simulink model "LKAS_AutoSave_DF_20211126_SW5"  (R2018b)
settings: Solver=FixedStepDiscrete  StartTime=0.0  StopTime=10.0  FixedStep=0.01  RelTol=1e-3
undefined symbols (not defined in the file): LKA_CarWidth, LKA_SampleTime, LKA_StrRatio_C, LKA_Veh2CamL_C, LKA_Veh2CamW_C, LKA_WhlBaseL_C, LL_CompSWA_C, LL_CrvtPrvwT_C, LL_DesDvt_C, LL_DvtComp_C, LL_DvtPrvwT_C, LL_DvtSpdDet_vDvtSpdMin_C, LL_HdAgExT_C, LL_HdAgPrvwT_C, LL_LAccMax_C, LL_LAccRMax_C, LL_LDW_EarliestWarnLine_C, LL_LDW_LatestWarnLine_C, LL_LDWS_SUPPRESS_HEADING, LL_LFClb_TFC_FfCtlRatio_C, LL_LFClb_TFC_KdBalance_C, LL_LFClb_TFC_KdMaxSWA_C, LL_LFClb_TFC_KdV1_C, LL_LFClb_TFC_KdV2_C, LL_LFClb_TFC_KdVehSpdLwr_C, LL_LFClb_TFC_KdVehSpdUpr_C, LL_LFClb_TFC_Ki_C, LL_LFClb_TFC_KiMaxSWA_C, LL_LFClb_TFC_Kp_C, LL_LFClb_TFC_KpKlat_C, LL_LFClb_TFC_KpV1_C, LL_LFClb_TFC_KpV2_C, LL_LFClb_TFC_KpVehSpdLwr_C, LL_LFClb_TFC_KpVehSpdUpr_C, LL_LFClb_TFC_PrvwT_C, LL_LKA_EarliestWarnLine_C, LL_LKA_LatestWarnLine_C, LL_LKAExPrcs_ExitC0Dvt, LL_LKAExPrcs_ExitC0Swt, LL_LKAExPrcs_tiExitTime1, LL_LKAExPrcs_tiExitTime2, LL_LKAExPrcs_tiExitTime3, LL_LKAS_OUT_OF_CONTROL_LAT_VEL, LL_LKAS_OUT_OF_CONTROL_TTLC, LL_LKASWASyn_M0, LL_LKASWASyn_M1, LL_LKASWASyn_M2, LL_LKASWASyn_M3K, LL_LKASWASyn_SWAaddMax, LL_LKASWASyn_T2, LL_LKASWASyn_tiTrqSwaRtTime, LL_LKASWASyn_tiTrqSwaTime, LL_LKASWASyn_TrqMax, LL_LKASWASyn_TrqSwaAddSwt, LL_LKASWASyn_TrqSwaRateDiff, LL_LSpdCompT_C, LL_lStpLngth_C, LL_MAX_DELAY_EPSSTAR_TIME, LL_MAX_DRIVER_TORQUE_DISABLE, LL_MAX_DRIVER_TORQUE_ENABLE ... (+38)
libraries: simulink x137, canmsglib x10, dspstat3 x3, simulink_extras x1
(part 1 of 13)
settings Model: Creator=hejr  LastModifiedBy=hejr
settings OptimizationCC: BlockReduction=off  DefaultParameterBehavior=Inlined  UseDivisionForNetSlopeComputation=on  UseFloatMulNetSlope=on  DefaultUnderspecifiedDataType=single  UseSpecifiedMinMax=on  InlineInvariantSignals=on  PassReuseOutputArgsAs=Individual arguments  ZeroExternalMemoryAtStartup=off  ZeroInternalMemoryAtStartup=off  NoFixptDivByZeroProtection=on  EfficientFloat2IntCast=on  LifeSpan=inf  OptimizeBlockOrder=speed  DifferentSizesBufferReuse=on
settings DebuggingCC: SignalInfNanChecking=error  ReadBeforeWriteMsg=EnableAllAsError  WriteAfterWriteMsg=EnableAllAsError  WriteAfterReadMsg=EnableAllAsError  IntegerOverflowMsg=error  ParameterTunabilityLossMsg=error  UniqueDataStoreMsg=error  AssertControl=DisableAll  NonBusSignalsTreatedAsBus=error  SFInvalidInputDataAccessInChartInitDiag=error  SFTransitionOutsideNaturalParentDiag=error  SFUnreachableExecutionPathDiag=error  SFUndirectedBroadcastEventsDiag=error  IntegerSaturationMsg=error
settings HardwareCC: ProdLongLongMode=on
settings ModelReferenceCC: UpdateModelReferenceTargets=IfOutOfDate
settings SFSimCC: SFSimEcho=off  CompileTimeRecursionLimit=0  EnableRuntimeRecursion=off  MATLABDynamicMemAlloc=off
settings RTWCC: SystemTargetFile=autosar.tlc  GenCodeOnly=on  TemplateMakefile=ert_default_tmf  Description=AUTOSAR  GenerateReport=on  BuildConfiguration=Faster Runs  IncludeHyperlinkInReport=on  LaunchReport=on  GenerateTraceInfo=on  GenerateTraceReport=on  GenerateTraceReportSl=on  GenerateTraceReportSf=on  GenerateTraceReportEml=on  GenerateCodeMetricsReport=on  GenerateCodeReplacementReport=on
settings CodeAppCC: ForceParamTrailComments=on  IgnoreCustomStorageClasses=off  OperatorAnnotations=on  SimulinkDataObjDesc=on  SFDataObjDesc=on  MATLABFcnDesc=on  InsertBlockDesc=on  StateflowObjectComments=on  MATLABSourceComments=on  EnableCustomComments=on  ReqsInCode=on
settings STFCustomTargetCC: TargetLangStandard=C99 (ISO)  MultiwordLength=256  ParMdlRefBuildCompliant=on  CompOptLevelCompliant=on  IncludeMdlTerminateFcn=off  CombineOutputUpdateFcns=on  CombineSignalStateStructs=on  SuppressErrorStatus=on  ERTCustomFileBanners=on  SupportNonFinite=off  SupportComplex=off  SupportContinuousTime=off  SupportNonInlinedSFcns=off  RemoveResetFunc=on  ParenthesesLevel=Maximum  CastingMode=Standards  MATLABClassNameForMDSCustomization=Simulink.SoftwareTarget.ERTCustomization  AutosarCompliant=on  UseToolchainInfoCompliant=on  LookupTableObjectStructAxisOrder=2,1,3,4,...  LUTObjectStructOrderEvenSpacing=Size,Table,Breakpoints  SystemTargetFile=autosar.tlc
settings ERTTargetCC: TargetLangStandard=C99 (ISO)  ConcurrentExecutionCompliant=off  IncludeMdlTerminateFcn=off  CombineSignalStateStructs=on  SuppressErrorStatus=on  SupportNonFinite=off  SupportComplex=off  ParenthesesLevel=Maximum  CastingMode=Standards  ModelStepFunctionPrototypeControlCompliant=off  CPPClassGenCompliant=off  AutosarCompliant=on  LookupTableObjectStructAxisOrder=2,1,3,4,...  LUTObjectStructOrderEvenSpacing=Size,Table,Breakpoints  GenerateASAP2=on  InlinedParameterPlacement=NonHierarchical  ERTCustomFileTemplate=example_file_process.tlc  EnableSignedLeftShifts=off  EnableSignedRightShifts=off

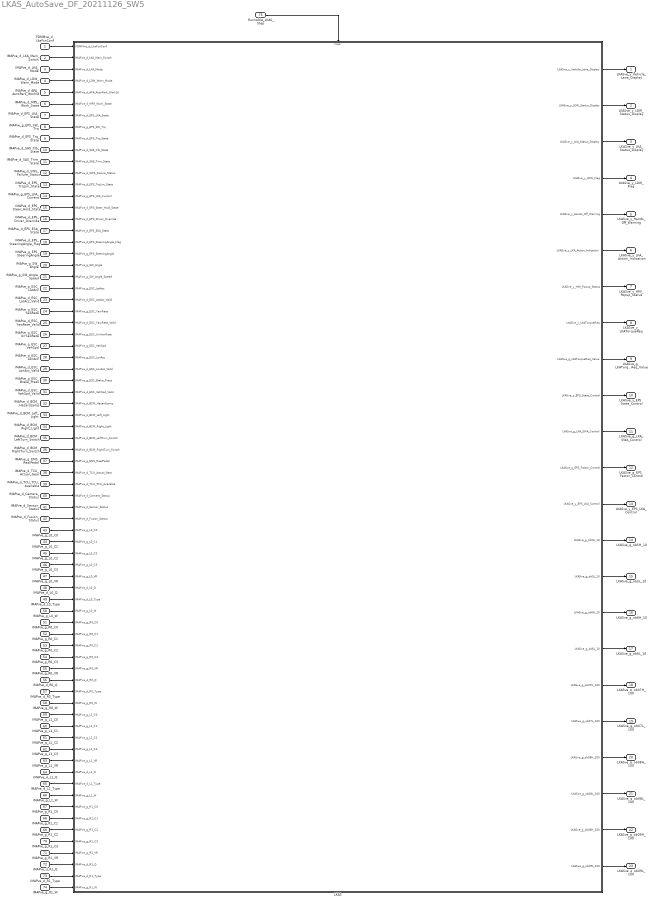
== system LKAS_AutoSave_DF_20211126_SW5 ==
  FDMMve_d_LkaFcnConf : Inport  OutDataTypeStr=UInt16  PortDimensions=1
  IMAPve_d_LKA_Main_Switch : Inport  Port=2  OutDataTypeStr=UInt16  PortDimensions=1
  IMAPve_d_LKA_Mode : Inport  Port=3  OutDataTypeStr=UInt16  PortDimensions=1
  IMAPve_d_LDW_Warn_Mode : Inport  Port=4  OutDataTypeStr=UInt16  PortDimensions=1
  IMAPve_d_APA_AutoPark_WorkSt : Inport  Port=5  OutDataTypeStr=UInt16  PortDimensions=1
  IMAPve_d_MP5_Work_State : Inport  Port=6  OutDataTypeStr=UInt16  PortDimensions=1
  IMAPve_d_EPS_LKA_State : Inport  Port=7  OutDataTypeStr=UInt16  PortDimensions=1
  IMAPve_g_EPS_SW_Trq : Inport  Port=8  OutDataTypeStr=T_M_Nm_Float32  PortDimensions=1
  IMAPve_d_EPS_Trq_State : Inport  Port=9  OutDataTypeStr=UInt16  PortDimensions=1
  IMAPve_d_SAS_Clb_State : Inport  Port=10  OutDataTypeStr=UInt16  PortDimensions=1
  IMAPve_d_SAS_Trim_State : Inport  Port=11  OutDataTypeStr=UInt16  PortDimensions=1
  IMAPve_d_SWS_Failure_Status : Inport  Port=12  OutDataTypeStr=UInt16  PortDimensions=1
  IMAPve_d_EPS_TrqLim_State : Inport  Port=13  OutDataTypeStr=UInt16  PortDimensions=1
  IMAPve_g_EPS_LKA_Current : Inport  Port=14  OutDataTypeStr=T_M_Nm_Float32  PortDimensions=1
  IMAPve_d_EPS_Steer_Hold_State : Inport  Port=15  OutDataTypeStr=UInt16  PortDimensions=1
  IMAPve_d_EPS_Driver_Override : Inport  Port=16  OutDataTypeStr=UInt16  PortDimensions=1
  IMAPve_d_EPS_ESA_State : Inport  Port=17  OutDataTypeStr=UInt16  PortDimensions=1
  IMAPve_d_EPS_SteeringAngle_Flag : Inport  Port=18  OutDataTypeStr=UInt16  PortDimensions=1
  IMAPve_g_EPS_SteeringAngle : Inport  Port=19  OutDataTypeStr=T_M_Nm_Float32  PortDimensions=1
  IMAPve_g_SW_Angle : Inport  Port=20  OutDataTypeStr=T_M_Nm_Float32  PortDimensions=1
  IMAPve_g_SW_Angle_Speed : Inport  Port=21  OutDataTypeStr=T_M_Nm_Float32  PortDimensions=1
  IMAPve_g_ESC_LatAcc : Inport  Port=22  OutDataTypeStr=T_M_Nm_Float32  PortDimensions=1
  IMAPve_d_ESC_LatAcc_Valid : Inport  Port=23  OutDataTypeStr=UInt16  PortDimensions=1
  IMAPve_g_ESC_YawRate : Inport  Port=24  OutDataTypeStr=T_M_Nm_Float32  PortDimensions=1
  IMAPve_d_ESC_YawRate_Valid : Inport  Port=25  OutDataTypeStr=UInt16  PortDimensions=1
  IMAPve_g_ESC_UnYawRate : Inport  Port=26  OutDataTypeStr=T_M_Nm_Float32  PortDimensions=1
  IMAPve_g_ESC_VehSpd : Inport  Port=27  OutDataTypeStr=T_M_Nm_Float32  PortDimensions=1
  IMAPve_g_ESC_LonAcc : Inport  Port=28  OutDataTypeStr=T_M_Nm_Float32  PortDimensions=1
  IMAPve_d_ESC_LonAcc_Valid : Inport  Port=29  OutDataTypeStr=UInt16  PortDimensions=1
  IMAPve_g_ESC_Brake_Press : Inport  Port=30  OutDataTypeStr=T_M_Nm_Float32  PortDimensions=1
  IMAPve_d_ESC_VehSpd_Valid : Inport  Port=31  OutDataTypeStr=UInt16  PortDimensions=1
  IMAPve_d_BCM_HazardLamp : Inport  Port=32  OutDataTypeStr=UInt16  PortDimensions=1
  IMAPve_d_BCM_Left_Light : Inport  Port=33  OutDataTypeStr=UInt16  PortDimensions=1
  IMAPve_d_BCM_Right_Light : Inport  Port=34  OutDataTypeStr=UInt16  PortDimensions=1
  IMAPve_d_BCM_LeftTurn_Switch : Inport  Port=35  OutDataTypeStr=UInt16  PortDimensions=1
  IMAPve_d_BCM_RightTurn_Switch : Inport  Port=36  OutDataTypeStr=UInt16  PortDimensions=1
  IMAPve_g_EMS_RealPedal : Inport  Port=37  OutDataTypeStr=T_M_Nm_Float32  PortDimensions=1
  IMAPve_d_TCU_Actual_Gear : Inport  Port=38  OutDataTypeStr=UInt16  PortDimensions=1
  IMAPve_d_TCU_TCU_Available : Inport  Port=39  OutDataTypeStr=UInt16  PortDimensions=1
  IMAPve_d_Camera_Status : Inport  Port=40  OutDataTypeStr=UInt16  PortDimensions=1
  IMAPve_d_Sensor_Status : Inport  Port=41  OutDataTypeStr=UInt16  PortDimensions=1
  IMAPve_d_Fusion_Status : Inport  Port=42  OutDataTypeStr=UInt16  PortDimensions=1
  IMAPve_g_L0_C0 : Inport  Port=43  OutDataTypeStr=T_M_Nm_Float32  PortDimensions=1
  IMAPve_g_L0_C1 : Inport  Port=44  OutDataTypeStr=T_M_Nm_Float32  PortDimensions=1
  IMAPve_g_L0_C2 : Inport  Port=45  OutDataTypeStr=T_M_Nm_Float32  PortDimensions=1
  IMAPve_g_L0_C3 : Inport  Port=46  OutDataTypeStr=T_M_Nm_Float32  PortDimensions=1
  IMAPve_g_L0_VR : Inport  Port=47  OutDataTypeStr=T_M_Nm_Float32  PortDimensions=1
  IMAPve_d_L0_Q : Inport  Port=48  OutDataTypeStr=UInt16  PortDimensions=1
  IMAPve_d_L0_Type : Inport  Port=49  OutDataTypeStr=UInt16  PortDimensions=1
  IMAPve_g_L0_W : Inport  Port=50  OutDataTypeStr=T_M_Nm_Float32  PortDimensions=1
  IMAPve_g_R0_C0 : Inport  Port=51  OutDataTypeStr=T_M_Nm_Float32  PortDimensions=1
  IMAPve_g_R0_C1 : Inport  Port=52  OutDataTypeStr=T_M_Nm_Float32  PortDimensions=1
  IMAPve_g_R0_C2 : Inport  Port=53  OutDataTypeStr=T_M_Nm_Float32  PortDimensions=1
  IMAPve_g_R0_C3 : Inport  Port=54  OutDataTypeStr=T_M_Nm_Float32  PortDimensions=1
  IMAPve_g_R0_VR : Inport  Port=55  OutDataTypeStr=T_M_Nm_Float32  PortDimensions=1
  IMAPve_d_R0_Q : Inport  Port=56  OutDataTypeStr=UInt16  PortDimensions=1
  IMAPve_d_R0_Type : Inport  Port=57  OutDataTypeStr=UInt16  PortDimensions=1
  IMAPve_g_R0_W : Inport  Port=58  OutDataTypeStr=T_M_Nm_Float32  PortDimensions=1
  IMAPve_g_L1_C0 : Inport  Port=59  OutDataTypeStr=T_M_Nm_Float32  PortDimensions=1
  IMAPve_g_L1_C1 : Inport  Port=60  OutDataTypeStr=T_M_Nm_Float32  PortDimensions=1
  IMAPve_g_L1_C2 : Inport  Port=61  OutDataTypeStr=T_M_Nm_Float32  PortDimensions=1
  IMAPve_g_L1_C3 : Inport  Port=62  OutDataTypeStr=T_M_Nm_Float32  PortDimensions=1
  IMAPve_g_L1_VR : Inport  Port=63  OutDataTypeStr=T_M_Nm_Float32  PortDimensions=1
  IMAPve_d_L1_Q : Inport  Port=64  OutDataTypeStr=UInt16  PortDimensions=1
  IMAPve_d_L1_Type : Inport  Port=65  OutDataTypeStr=UInt16  PortDimensions=1
  IMAPve_g_L1_W : Inport  Port=66  OutDataTypeStr=T_M_Nm_Float32  PortDimensions=1
  IMAPve_g_R1_C0 : Inport  Port=67  OutDataTypeStr=T_M_Nm_Float32  PortDimensions=1
  IMAPve_g_R1_C1 : Inport  Port=68  OutDataTypeStr=T_M_Nm_Float32  PortDimensions=1
  IMAPve_g_R1_C2 : Inport  Port=69  OutDataTypeStr=T_M_Nm_Float32  PortDimensions=1
  IMAPve_g_R1_C3 : Inport  Port=70  OutDataTypeStr=T_M_Nm_Float32  PortDimensions=1
  IMAPve_g_R1_VR : Inport  Port=71  OutDataTypeStr=T_M_Nm_Float32  PortDimensions=1
  IMAPve_d_R1_Q : Inport  Port=72  OutDataTypeStr=UInt16  PortDimensions=1
  IMAPve_d_R1_Type : Inport  Port=73  OutDataTypeStr=UInt16  PortDimensions=1
  IMAPve_g_R1_W : Inport  Port=74  OutDataTypeStr=T_M_Nm_Float32  PortDimensions=1
  Runnable_LKAS_Step : Inport  Port=75  SampleTime=0.01  OutputFunctionCall=on
  LKAS : Subsystem  TreatAsAtomicUnit=on
  LKASve_y_Vehicle_Lane_Display : Outport  OutDataTypeStr=UInt8  PortDimensions=1
  LKASve_y_LDW_Status_Display : Outport  Port=2  OutDataTypeStr=UInt8  PortDimensions=1
  LKASve_y_LKA_Status_Display : Outport  Port=3  OutDataTypeStr=UInt8  PortDimensions=1
  LKASve_y_LDW_Flag : Outport  Port=4  OutDataTypeStr=UInt8  PortDimensions=1
  LKASve_y_Hands_Off_Warning : Outport  Port=5  OutDataTypeStr=UInt8  PortDimensions=1
  LKASve_y_LKA_Action_Indication : Outport  Port=6  OutDataTypeStr=UInt8  PortDimensions=1
  LKASve_y_HMI_Popup_Status : Outport  Port=7  OutDataTypeStr=UInt8  PortDimensions=1
  LKASve_y_LKATorqueReq : Outport  Port=8  OutDataTypeStr=UInt8  PortDimensions=1
  LKASve_g_LKATorqueReq_Value : Outport  Port=9  OutDataTypeStr=T_M_Nm_Float32  PortDimensions=1
  LKASve_y_EPS_State_Control : Outport  Port=10  OutDataTypeStr=UInt8  PortDimensions=1
  LKASve_g_LKA_SWA_Control : Outport  Port=11  OutDataTypeStr=T_M_Nm_Float32  PortDimensions=1
  LKASve_g_EPS_Factor_Control : Outport  Port=12  OutDataTypeStr=T_M_Nm_Float32  PortDimensions=1
  LKASve_y_EPS_LKA_Control : Outport  Port=13  OutDataTypeStr=UInt8  PortDimensions=1
  LKASve_g_ob5H_10 : Outport  Port=14  OutDataTypeStr=UInt32  PortDimensions=1
  LKASve_g_ob5L_10 : Outport  Port=15  OutDataTypeStr=UInt32  PortDimensions=1
  LKASve_g_ob6H_10 : Outport  Port=16  OutDataTypeStr=UInt32  PortDimensions=1
  LKASve_g_ob6L_10 : Outport  Port=17  OutDataTypeStr=UInt32  PortDimensions=1
  LKASve_g_ob07H_100 : Outport  Port=18  OutDataTypeStr=UInt32  PortDimensions=1
  LKASve_g_ob07L_100 : Outport  Port=19  OutDataTypeStr=UInt32  PortDimensions=1
  LKASve_g_ob08H_100 : Outport  Port=20  OutDataTypeStr=UInt32  PortDimensions=1
  LKASve_g_ob08L_100 : Outport  Port=21  OutDataTypeStr=UInt32  PortDimensions=1
  LKASve_g_ob09H_100 : Outport  Port=22  OutDataTypeStr=UInt32  PortDimensions=1
  LKASve_g_ob09L_100 : Outport  Port=23  OutDataTypeStr=UInt32  PortDimensions=1
  wires:
  FDMMve_d_LkaFcnConf/1 -> LKAS/1(FDMMve_d_LkaFcnConf)
  IMAPve_d_LKA_Main_Switch/1 -> LKAS/2(IMAPve_d_LKA_Main_Switch)
  IMAPve_d_LKA_Mode/1 -> LKAS/3(IMAPve_d_LKA_Mode)
  IMAPve_d_LDW_Warn_Mode/1 -> LKAS/4(IMAPve_d_LDW_Warn_Mode)
  IMAPve_d_APA_AutoPark_WorkSt/1 -> LKAS/5(IMAPve_d_APA_AutoPark_WorkSt)
  IMAPve_d_MP5_Work_State/1 -> LKAS/6(IMAPve_d_MP5_Work_State)
  IMAPve_d_EPS_LKA_State/1 -> LKAS/7(IMAPve_d_EPS_LKA_State)
  IMAPve_g_EPS_SW_Trq/1 -> LKAS/8(IMAPve_g_EPS_SW_Trq)
  IMAPve_d_EPS_Trq_State/1 -> LKAS/9(IMAPve_d_EPS_Trq_State)
  IMAPve_d_SAS_Clb_State/1 -> LKAS/10(IMAPve_d_SAS_Clb_State)
  IMAPve_d_SAS_Trim_State/1 -> LKAS/11(IMAPve_d_SAS_Trim_State)
  IMAPve_d_SWS_Failure_Status/1 -> LKAS/12(IMAPve_d_SWS_Failure_Status)
  IMAPve_d_EPS_TrqLim_State/1 -> LKAS/13(IMAPve_d_EPS_TrqLim_State)
  IMAPve_g_EPS_LKA_Current/1 -> LKAS/14(IMAPve_g_EPS_LKA_Current)
  IMAPve_d_EPS_Steer_Hold_State/1 -> LKAS/15(IMAPve_d_EPS_Steer_Hold_State)
  IMAPve_d_EPS_Driver_Override/1 -> LKAS/16(IMAPve_d_EPS_Driver_Override)
  IMAPve_d_EPS_ESA_State/1 -> LKAS/17(IMAPve_d_EPS_ESA_State)
  IMAPve_d_EPS_SteeringAngle_Flag/1 -> LKAS/18(IMAPve_d_EPS_SteeringAngle_Flag)
  IMAPve_g_EPS_SteeringAngle/1 -> LKAS/19(IMAPve_g_EPS_SteeringAngle)
  IMAPve_g_SW_Angle/1 -> LKAS/20(IMAPve_g_SW_Angle)
  IMAPve_g_SW_Angle_Speed/1 -> LKAS/21(IMAPve_g_SW_Angle_Speed)
  IMAPve_g_ESC_LatAcc/1 -> LKAS/22(IMAPve_g_ESC_LatAcc)
  IMAPve_d_ESC_LatAcc_Valid/1 -> LKAS/23(IMAPve_d_ESC_LatAcc_Valid)
  IMAPve_g_ESC_YawRate/1 -> LKAS/24(IMAPve_g_ESC_YawRate)
  IMAPve_d_ESC_YawRate_Valid/1 -> LKAS/25(IMAPve_d_ESC_YawRate_Valid)
  IMAPve_g_ESC_UnYawRate/1 -> LKAS/26(IMAPve_g_ESC_UnYawRate)
  IMAPve_g_ESC_VehSpd/1 -> LKAS/27(IMAPve_g_ESC_VehSpd)
  IMAPve_g_ESC_LonAcc/1 -> LKAS/28(IMAPve_g_ESC_LonAcc)
  IMAPve_d_ESC_LonAcc_Valid/1 -> LKAS/29(IMAPve_d_ESC_LonAcc_Valid)
  IMAPve_g_ESC_Brake_Press/1 -> LKAS/30(IMAPve_g_ESC_Brake_Press)
  IMAPve_d_ESC_VehSpd_Valid/1 -> LKAS/31(IMAPve_d_ESC_VehSpd_Valid)
  IMAPve_d_BCM_HazardLamp/1 -> LKAS/32(IMAPve_d_BCM_HazardLamp)
  IMAPve_d_BCM_Left_Light/1 -> LKAS/33(IMAPve_d_BCM_Left_Light)
  IMAPve_d_BCM_Right_Light/1 -> LKAS/34(IMAPve_d_BCM_Right_Light)
  IMAPve_d_BCM_LeftTurn_Switch/1 -> LKAS/35(IMAPve_d_BCM_LeftTurn_Switch)
  IMAPve_d_BCM_RightTurn_Switch/1 -> LKAS/36(IMAPve_d_BCM_RightTurn_Switch)
  IMAPve_g_EMS_RealPedal/1 -> LKAS/37(IMAPve_g_EMS_RealPedal)
  IMAPve_d_TCU_Actual_Gear/1 -> LKAS/38(IMAPve_d_TCU_Actual_Gear)
  IMAPve_d_TCU_TCU_Available/1 -> LKAS/39(IMAPve_d_TCU_TCU_Available)
  IMAPve_d_Camera_Status/1 -> LKAS/40(IMAPve_d_Camera_Status)
  IMAPve_d_Sensor_Status/1 -> LKAS/41(IMAPve_d_Sensor_Status)
  IMAPve_d_Fusion_Status/1 -> LKAS/42(IMAPve_d_Fusion_Status)
  IMAPve_g_L0_C0/1 -> LKAS/43(IMAPve_g_L0_C0)
  IMAPve_g_L0_C1/1 -> LKAS/44(IMAPve_g_L0_C1)
  IMAPve_g_L0_C2/1 -> LKAS/45(IMAPve_g_L0_C2)
  IMAPve_g_L0_C3/1 -> LKAS/46(IMAPve_g_L0_C3)
  IMAPve_g_L0_VR/1 -> LKAS/47(IMAPve_g_L0_VR)
  IMAPve_d_L0_Q/1 -> LKAS/48(IMAPve_d_L0_Q)
  IMAPve_d_L0_Type/1 -> LKAS/49(IMAPve_d_L0_Type)
  IMAPve_g_L0_W/1 -> LKAS/50(IMAPve_g_L0_W)
  IMAPve_g_R0_C0/1 -> LKAS/51(IMAPve_g_R0_C0)
  IMAPve_g_R0_C1/1 -> LKAS/52(IMAPve_g_R0_C1)
  IMAPve_g_R0_C2/1 -> LKAS/53(IMAPve_g_R0_C2)
  IMAPve_g_R0_C3/1 -> LKAS/54(IMAPve_g_R0_C3)
  IMAPve_g_R0_VR/1 -> LKAS/55(IMAPve_g_R0_VR)
  IMAPve_d_R0_Q/1 -> LKAS/56(IMAPve_d_R0_Q)
  IMAPve_d_R0_Type/1 -> LKAS/57(IMAPve_d_R0_Type)
  IMAPve_g_R0_W/1 -> LKAS/58(IMAPve_g_R0_W)
  IMAPve_g_L1_C0/1 -> LKAS/59(IMAPve_g_L1_C0)
  IMAPve_g_L1_C1/1 -> LKAS/60(IMAPve_g_L1_C1)
  IMAPve_g_L1_C2/1 -> LKAS/61(IMAPve_g_L1_C2)
  IMAPve_g_L1_C3/1 -> LKAS/62(IMAPve_g_L1_C3)
  IMAPve_g_L1_VR/1 -> LKAS/63(IMAPve_g_L1_VR)
  IMAPve_d_L1_Q/1 -> LKAS/64(IMAPve_d_L1_Q)
  IMAPve_d_L1_Type/1 -> LKAS/65(IMAPve_d_L1_Type)
  IMAPve_g_L1_W/1 -> LKAS/66(IMAPve_g_L1_W)
  IMAPve_g_R1_C0/1 -> LKAS/67(IMAPve_g_R1_C0)
  IMAPve_g_R1_C1/1 -> LKAS/68(IMAPve_g_R1_C1)
  IMAPve_g_R1_C2/1 -> LKAS/69(IMAPve_g_R1_C2)
  IMAPve_g_R1_C3/1 -> LKAS/70(IMAPve_g_R1_C3)
  IMAPve_g_R1_VR/1 -> LKAS/71(IMAPve_g_R1_VR)
  IMAPve_d_R1_Q/1 -> LKAS/72(IMAPve_d_R1_Q)
  IMAPve_d_R1_Type/1 -> LKAS/73(IMAPve_d_R1_Type)
  IMAPve_g_R1_W/1 -> LKAS/74(IMAPve_g_R1_W)
  Runnable_LKAS_Step/1 -> LKAS/Trigger
  LKAS/1(LKASve_y_Vehicle_Lane_Display) -> LKASve_y_Vehicle_Lane_Display/1
  LKAS/2(LKASve_y_LDW_Status_Display) -> LKASve_y_LDW_Status_Display/1
  LKAS/3(LKASve_y_LKA_Status_Display) -> LKASve_y_LKA_Status_Display/1
  LKAS/4(LKASve_y_LDW_Flag) -> LKASve_y_LDW_Flag/1
  LKAS/5(LKASve_y_Hands_Off_Warning) -> LKASve_y_Hands_Off_Warning/1
  LKAS/6(LKASve_y_LKA_Action_Indication) -> LKASve_y_LKA_Action_Indication/1
  LKAS/7(LKASve_y_HMI_Popup_Status) -> LKASve_y_HMI_Popup_Status/1
  LKAS/8(LKASve_y_LKATorqueReq) -> LKASve_y_LKATorqueReq/1
  LKAS/9(LKASve_g_LKATorqueReq_Value) -> LKASve_g_LKATorqueReq_Value/1
  LKAS/10(LKASve_y_EPS_State_Control) -> LKASve_y_EPS_State_Control/1
  LKAS/11(LKASve_g_LKA_SWA_Control) -> LKASve_g_LKA_SWA_Control/1
  LKAS/12(LKASve_g_EPS_Factor_Control) -> LKASve_g_EPS_Factor_Control/1
  LKAS/13(LKASve_y_EPS_LKA_Control) -> LKASve_y_EPS_LKA_Control/1
  LKAS/14(LKASve_g_ob5H_10) -> LKASve_g_ob5H_10/1
  LKAS/15(LKASve_g_ob5L_10) -> LKASve_g_ob5L_10/1
  LKAS/16(LKASve_g_ob6H_10) -> LKASve_g_ob6H_10/1
  LKAS/17(LKASve_g_ob6L_10) -> LKASve_g_ob6L_10/1
  LKAS/18(LKASve_g_ob07H_100) -> LKASve_g_ob07H_100/1
  LKAS/19(LKASve_g_ob07L_100) -> LKASve_g_ob07L_100/1
  LKAS/20(LKASve_g_ob08H_100) -> LKASve_g_ob08H_100/1
  LKAS/21(LKASve_g_ob08L_100) -> LKASve_g_ob08L_100/1
  LKAS/22(LKASve_g_ob09H_100) -> LKASve_g_ob09H_100/1
  LKAS/23(LKASve_g_ob09L_100) -> LKASve_g_ob09L_100/1

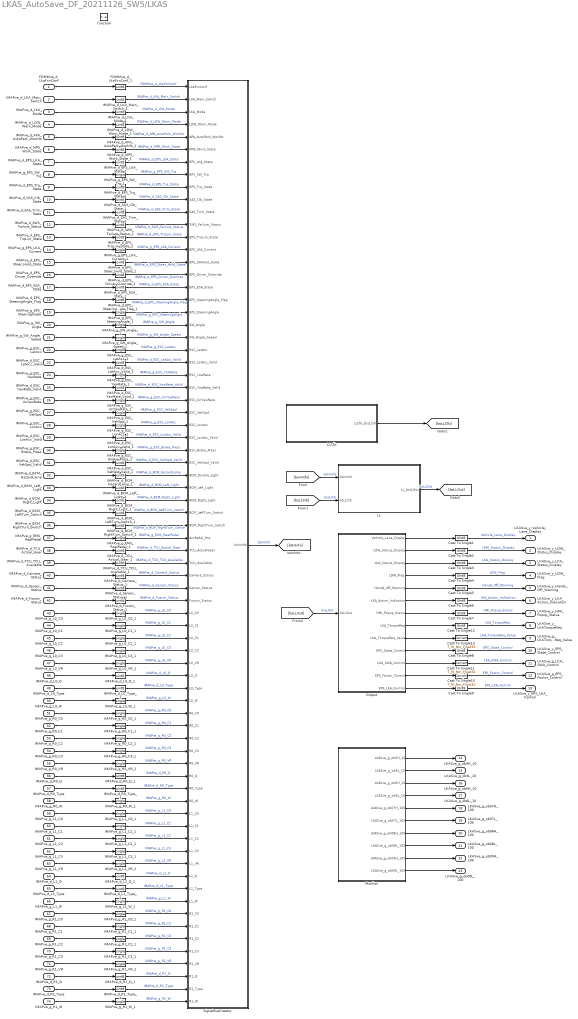
== system LKAS_AutoSave_DF_20211126_SW5/LKAS ==
  FDMMve_d_LkaFcnConf : Inport
  IMAPve_d_LKA_Main_Switch : Inport  Port=2
  IMAPve_d_LKA_Mode : Inport  Port=3
  IMAPve_d_LDW_Warn_Mode : Inport  Port=4
  IMAPve_d_APA_AutoPark_WorkSt : Inport  Port=5
  IMAPve_d_MP5_Work_State : Inport  Port=6
  IMAPve_d_EPS_LKA_State : Inport  Port=7
  IMAPve_g_EPS_SW_Trq : Inport  Port=8
  IMAPve_d_EPS_Trq_State : Inport  Port=9
  IMAPve_d_SAS_Clb_State : Inport  Port=10
  IMAPve_d_SAS_Trim_State : Inport  Port=11
  IMAPve_d_SWS_Failure_Status : Inport  Port=12
  IMAPve_d_EPS_TrqLim_State : Inport  Port=13
  IMAPve_g_EPS_LKA_Current : Inport  Port=14
  IMAPve_d_EPS_Steer_Hold_State : Inport  Port=15
  IMAPve_d_EPS_Driver_Override : Inport  Port=16
  IMAPve_d_EPS_ESA_State : Inport  Port=17
  IMAPve_d_EPS_SteeringAngle_Flag : Inport  Port=18
  IMAPve_g_EPS_SteeringAngle : Inport  Port=19
  IMAPve_g_SW_Angle : Inport  Port=20
  IMAPve_g_SW_Angle_Speed : Inport  Port=21
  IMAPve_g_ESC_LatAcc : Inport  Port=22
  IMAPve_d_ESC_LatAcc_Valid : Inport  Port=23
  IMAPve_g_ESC_YawRate : Inport  Port=24
  IMAPve_d_ESC_YawRate_Valid : Inport  Port=25
  IMAPve_g_ESC_UnYawRate : Inport  Port=26
  IMAPve_g_ESC_VehSpd : Inport  Port=27
  IMAPve_g_ESC_LonAcc : Inport  Port=28
  IMAPve_d_ESC_LonAcc_Valid : Inport  Port=29
  IMAPve_g_ESC_Brake_Press : Inport  Port=30
  IMAPve_d_ESC_VehSpd_Valid : Inport  Port=31
  IMAPve_d_BCM_HazardLamp : Inport  Port=32
  IMAPve_d_BCM_Left_Light : Inport  Port=33
  IMAPve_d_BCM_Right_Light : Inport  Port=34
  IMAPve_d_BCM_LeftTurn_Switch : Inport  Port=35
  IMAPve_d_BCM_RightTurn_Switch : Inport  Port=36
  IMAPve_g_EMS_RealPedal : Inport  Port=37
  IMAPve_d_TCU_Actual_Gear : Inport  Port=38
  IMAPve_d_TCU_TCU_Available : Inport  Port=39
  IMAPve_d_Camera_Status : Inport  Port=40
  IMAPve_d_Sensor_Status : Inport  Port=41
  IMAPve_d_Fusion_Status : Inport  Port=42
  IMAPve_g_L0_C0 : Inport  Port=43
  IMAPve_g_L0_C1 : Inport  Port=44
  IMAPve_g_L0_C2 : Inport  Port=45
  IMAPve_g_L0_C3 : Inport  Port=46
  IMAPve_g_L0_VR : Inport  Port=47
  IMAPve_d_L0_Q : Inport  Port=48
  IMAPve_d_L0_Type : Inport  Port=49
  IMAPve_g_L0_W : Inport  Port=50
  IMAPve_g_R0_C0 : Inport  Port=51
  IMAPve_g_R0_C1 : Inport  Port=52
  IMAPve_g_R0_C2 : Inport  Port=53
  IMAPve_g_R0_C3 : Inport  Port=54
  IMAPve_g_R0_VR : Inport  Port=55
  IMAPve_d_R0_Q : Inport  Port=56
  IMAPve_d_R0_Type : Inport  Port=57
  IMAPve_g_R0_W : Inport  Port=58
  IMAPve_g_L1_C0 : Inport  Port=59
  IMAPve_g_L1_C1 : Inport  Port=60
  IMAPve_g_L1_C2 : Inport  Port=61
  IMAPve_g_L1_C3 : Inport  Port=62
  IMAPve_g_L1_VR : Inport  Port=63
  IMAPve_d_L1_Q : Inport  Port=64
  IMAPve_d_L1_Type : Inport  Port=65
  IMAPve_g_L1_W : Inport  Port=66
  IMAPve_g_R1_C0 : Inport  Port=67
  IMAPve_g_R1_C1 : Inport  Port=68
  IMAPve_g_R1_C2 : Inport  Port=69
  IMAPve_g_R1_C3 : Inport  Port=70
  IMAPve_g_R1_VR : Inport  Port=71
  IMAPve_d_R1_Q : Inport  Port=72
  IMAPve_d_R1_Type : Inport  Port=73
  IMAPve_g_R1_W : Inport  Port=74
  function : TriggerPort  TriggerType=function-call  VariantControl=Variant  SampleTimeType=periodic  SampleTime=-1
  Cast To Single{1..9,12} (10 alike) : DataTypeConversion  OutDataTypeStr=UInt8
  Cast To Single10 : DataTypeConversion  OutDataTypeStr=T_M_Nm_Float32
  Cast To Single11 : DataTypeConversion  OutDataTypeStr=T_M_Nm_Float32
  Cast To Single13 : DataTypeConversion  OutDataTypeStr=T_M_Nm_Float32
  FDMMve_d_LkaFcnConf_1 : DataTypeConversion  OutDataTypeStr=uint8
  IMAPve_d_APA_AutoPark_WorkSt_1 : DataTypeConversion  OutDataTypeStr=uint8
  IMAPve_d_BCM_HazardLamp_1 : DataTypeConversion  OutDataTypeStr=uint8
  IMAPve_d_BCM_LeftTurn_Switch_1 : DataTypeConversion  OutDataTypeStr=uint8
  IMAPve_d_BCM_Left_Light_1 : DataTypeConversion  OutDataTypeStr=uint8
  IMAPve_d_BCM_RightTurn_Switch_1 : DataTypeConversion  OutDataTypeStr=uint8
  IMAPve_d_BCM_Right_Light_1 : DataTypeConversion  OutDataTypeStr=uint8
  IMAPve_d_Camera_Status_1 : DataTypeConversion  OutDataTypeStr=uint8
  IMAPve_d_EPS_Driver_Override_1 : DataTypeConversion  OutDataTypeStr=uint8
  IMAPve_d_EPS_ESA_State_1 : DataTypeConversion  OutDataTypeStr=uint8
  IMAPve_d_EPS_LKA_State_1 : DataTypeConversion  OutDataTypeStr=uint8
  IMAPve_d_EPS_Steer_Hold_State_1 : DataTypeConversion  OutDataTypeStr=uint8
  IMAPve_d_EPS_SteeringAngle_Flag_1 : DataTypeConversion  OutDataTypeStr=uint8
  IMAPve_d_EPS_TrqLim_State_1 : DataTypeConversion  OutDataTypeStr=uint8
  IMAPve_d_EPS_Trq_State_1 : DataTypeConversion  OutDataTypeStr=uint8
  IMAPve_d_ESC_LatAcc_Valid_1 : DataTypeConversion  OutDataTypeStr=uint8
  IMAPve_d_ESC_LonAcc_Valid_1 : DataTypeConversion  OutDataTypeStr=uint8
  IMAPve_d_ESC_VehSpd_Valid_1 : DataTypeConversion  OutDataTypeStr=uint8
  IMAPve_d_ESC_YawRate_Valid_1 : DataTypeConversion  OutDataTypeStr=uint8
  IMAPve_d_Fusion_Status_1 : DataTypeConversion  OutDataTypeStr=uint8
  IMAPve_d_L0_Q_1 : DataTypeConversion  OutDataTypeStr=uint8
  IMAPve_d_L0_Type_1 : DataTypeConversion  OutDataTypeStr=uint8
  IMAPve_d_L1_Q_1 : DataTypeConversion  OutDataTypeStr=uint8
  IMAPve_d_L1_Type_1 : DataTypeConversion  OutDataTypeStr=uint8
  IMAPve_d_LDW_Warn_Mode_1 : DataTypeConversion  OutDataTypeStr=uint8
  IMAPve_d_LKA_Main_Switch_1 : DataTypeConversion  OutDataTypeStr=uint8
  IMAPve_d_LKA_Mode_1 : DataTypeConversion  OutDataTypeStr=uint8
  IMAPve_d_MP5_Work_State_1 : DataTypeConversion  OutDataTypeStr=uint8
  IMAPve_d_R0_Q_1 : DataTypeConversion  OutDataTypeStr=uint8
  IMAPve_d_R0_Type_1 : DataTypeConversion  OutDataTypeStr=uint8
  IMAPve_d_R1_Q_1 : DataTypeConversion  OutDataTypeStr=uint8
  IMAPve_d_R1_Type_1 : DataTypeConversion  OutDataTypeStr=uint8
  IMAPve_d_SAS_Clb_State_1 : DataTypeConversion  OutDataTypeStr=uint8
  IMAPve_d_SAS_Trim_State_1 : DataTypeConversion  OutDataTypeStr=uint8
  IMAPve_d_SWS_Failure_Status_1 : DataTypeConversion  OutDataTypeStr=uint8
  IMAPve_d_Sensor_Status_1 : DataTypeConversion  OutDataTypeStr=uint8
  IMAPve_d_TCU_Actual_Gear_1 : DataTypeConversion  OutDataTypeStr=uint8
  IMAPve_d_TCU_TCU_Available_1 : DataTypeConversion  OutDataTypeStr=uint8
  IMAPve_g_EMS_RealPedal_1 : DataTypeConversion  OutDataTypeStr=single
  IMAPve_g_EPS_LKA_Current_1 : DataTypeConversion  OutDataTypeStr=single
  IMAPve_g_EPS_SW_Trq_1 : DataTypeConversion  OutDataTypeStr=single
  IMAPve_g_EPS_SteeringAngle_1 : DataTypeConversion  OutDataTypeStr=single
  IMAPve_g_ESC_Brake_Press_1 : DataTypeConversion  OutDataTypeStr=single
  IMAPve_g_ESC_LatAcc_1 : DataTypeConversion  OutDataTypeStr=single
  IMAPve_g_ESC_LonAcc_1 : DataTypeConversion  OutDataTypeStr=single
  IMAPve_g_ESC_UnYawRate_1 : DataTypeConversion  OutDataTypeStr=single
  IMAPve_g_ESC_VehSpd_1 : DataTypeConversion  OutDataTypeStr=single
  IMAPve_g_ESC_YawRate_1 : DataTypeConversion  OutDataTypeStr=single
  IMAPve_g_L0_C0_1 : DataTypeConversion  OutDataTypeStr=single
  IMAPve_g_L0_C1_1 : DataTypeConversion  OutDataTypeStr=single
  IMAPve_g_L0_C2_1 : DataTypeConversion  OutDataTypeStr=single
  IMAPve_g_L0_C3_1 : DataTypeConversion  OutDataTypeStr=single
  IMAPve_g_L0_VR_1 : DataTypeConversion  OutDataTypeStr=single
  IMAPve_g_L0_W_1 : DataTypeConversion  OutDataTypeStr=single
  IMAPve_g_L1_C0_1 : DataTypeConversion  OutDataTypeStr=single
  IMAPve_g_L1_C1_1 : DataTypeConversion  OutDataTypeStr=single
  IMAPve_g_L1_C2_1 : DataTypeConversion  OutDataTypeStr=single
  IMAPve_g_L1_C3_1 : DataTypeConversion  OutDataTypeStr=single
  IMAPve_g_L1_VR_1 : DataTypeConversion  OutDataTypeStr=single
  IMAPve_g_L1_W_1 : DataTypeConversion  OutDataTypeStr=single
  IMAPve_g_R0_C0_1 : DataTypeConversion  OutDataTypeStr=single
  IMAPve_g_R0_C1_1 : DataTypeConversion  OutDataTypeStr=single
  IMAPve_g_R0_C2_1 : DataTypeConversion  OutDataTypeStr=single
  IMAPve_g_R0_C3_1 : DataTypeConversion  OutDataTypeStr=single
  IMAPve_g_R0_VR_1 : DataTypeConversion  OutDataTypeStr=single
  IMAPve_g_R0_W_1 : DataTypeConversion  OutDataTypeStr=single
  IMAPve_g_R1_C0_1 : DataTypeConversion  OutDataTypeStr=single
  IMAPve_g_R1_C1_1 : DataTypeConversion  OutDataTypeStr=single
  IMAPve_g_R1_C2_1 : DataTypeConversion  OutDataTypeStr=single
  IMAPve_g_R1_C3_1 : DataTypeConversion  OutDataTypeStr=single
  IMAPve_g_R1_VR_1 : DataTypeConversion  OutDataTypeStr=single
  IMAPve_g_R1_W_1 : DataTypeConversion  OutDataTypeStr=single
  IMAPve_g_SW_Angle_1 : DataTypeConversion  OutDataTypeStr=single
  IMAPve_g_SW_Angle_Speed_1 : DataTypeConversion  OutDataTypeStr=single
  LL : Subsystem
  LLClb : Subsystem
  Monitor : Subsystem  SystemSampleTime=0.01
  Output : Subsystem
  SignalBusCreator : Subsystem
  LKASve_y_Vehicle_Lane_Display : Outport
  LKASve_y_LDW_Status_Display : Outport  Port=2
  LKASve_y_LKA_Status_Display : Outport  Port=3
  LKASve_y_LDW_Flag : Outport  Port=4
  LKASve_y_Hands_Off_Warning : Outport  Port=5
  LKASve_y_LKA_Action_Indication : Outport  Port=6
  LKASve_y_HMI_Popup_Status : Outport  Port=7
  LKASve_y_LKATorqueReq : Outport  Port=8
  LKASve_g_LKATorqueReq_Value : Outport  Port=9
  LKASve_y_EPS_State_Control : Outport  Port=10
  LKASve_g_LKA_SWA_Control : Outport  Port=11
  LKASve_g_EPS_Factor_Control : Outport  Port=12
  LKASve_y_EPS_LKA_Control : Outport  Port=13
  LKASve_g_ob5H_10 : Outport  Port=14
  LKASve_g_ob5L_10 : Outport  Port=15
  LKASve_g_ob6H_10 : Outport  Port=16
  LKASve_g_ob6L_10 : Outport  Port=17
  LKASve_g_ob07H_100 : Outport  Port=18
  LKASve_g_ob07L_100 : Outport  Port=19
  LKASve_g_ob08H_100 : Outport  Port=20
  LKASve_g_ob08L_100 : Outport  Port=21
  LKASve_g_ob09H_100 : Outport  Port=22
  LKASve_g_ob09L_100 : Outport  Port=23
  wires:
  Cast To Single9/1 -> LKASve_y_EPS_LKA_Control/1  "EPS_LKA_Control"
  Cast To Single10/1 -> LKASve_g_EPS_Factor_Control/1  "EPS_Factor_Control"
  Cast To Single11/1 -> LKASve_g_LKA_SWA_Control/1  "LKA_SWA_Control"
  Cast To Single8/1 -> LKASve_y_EPS_State_Control/1  "EPS_State_Control"
  Cast To Single13/1 -> LKASve_g_LKATorqueReq_Value/1  "LKA_TorqueReq_Value"
  Cast To Single12/1 -> LKASve_y_LKATorqueReq/1  "LKA_TorqueReq"
  Cast To Single7/1 -> LKASve_y_HMI_Popup_Status/1  "HMI_Popup_Status"
  Cast To Single6/1 -> LKASve_y_LKA_Action_Indication/1  "LKA_Action_Indication"
  Cast To Single5/1 -> LKASve_y_Hands_Off_Warning/1  "Hands_Off_Warning"
  Cast To Single4/1 -> LKASve_y_LDW_Flag/1  "LDW_Flag"
  Cast To Single3/1 -> LKASve_y_LKA_Status_Display/1  "LKA_Status_Display"
  Cast To Single2/1 -> LKASve_y_LDW_Status_Display/1  "LDW_Status_Display"
  Cast To Single1/1 -> LKASve_y_Vehicle_Lane_Display/1  "Vehicle_Lane_Display"
  Output/13(EPS_LKA_Control) -> Cast To Single9/1
  Output/12(EPS_Factor_Control) -> Cast To Single10/1
  Output/11(LKA_SWA_Control) -> Cast To Single11/1
  Output/10(EPS_State_Control) -> Cast To Single8/1
  Output/9(LKA_TorqueReq_Value) -> Cast To Single13/1
  Output/8(LKA_TorqueReq) -> Cast To Single12/1
  Output/7(HMI_Popup_Status) -> Cast To Single7/1
  Output/6(LKA_Action_Indication) -> Cast To Single6/1
  Output/5(Hands_Off_Warning) -> Cast To Single5/1
  Output/4(LDW_Flag) -> Cast To Single4/1
  Output/3(LKA_Status_Display) -> Cast To Single3/1
  Output/2(LDW_Status_Display) -> Cast To Single2/1
  Output/1(Vehicle_Lane_Display) -> Cast To Single1/1
  Monitor/2(LKASve_g_ob5L_10) -> LKASve_g_ob5L_10/1
  [bsInInfo] -> LL/1(bsInInfo)  "bsInInfo"
  Monitor/5(LKASve_g_ob07H_100) -> LKASve_g_ob07H_100/1
  Monitor/10(LKASve_g_ob09L_100) -> LKASve_g_ob09L_100/1
  Monitor/4(LKASve_g_ob6L_10) -> LKASve_g_ob6L_10/1
  SignalBusCreator/1(bsInInfo) -> [bsInInfo]  "bsInInfo"
  LLClb/1(LLClb_bsLLClb) -> [bsLLClb]
  LL/1(LL_bsLLOut) -> [bsLLOut]  "bsLLOut"
  [bsLLClb] -> LL/2(bsLLClb)  "bsLLClb"
  Monitor/3(LKASve_g_ob6H_10) -> LKASve_g_ob6H_10/1
  Monitor/6(LKASve_g_ob07L_100) -> LKASve_g_ob07L_100/1
  [bsLLOut] -> Output/1(bsLLOut)  "bsLLOut"
  Monitor/7(LKASve_g_ob08H_100) -> LKASve_g_ob08H_100/1
  Monitor/8(LKASve_g_ob08L_100) -> LKASve_g_ob08L_100/1
  Monitor/9(LKASve_g_ob09H_100) -> LKASve_g_ob09H_100/1
  Monitor/1(LKASve_g_ob5H_10) -> LKASve_g_ob5H_10/1
  IMAPve_g_R1_W_1/1 -> SignalBusCreator/74(R1_W)  "IMAPve_g_R1_W"
  IMAPve_g_R1_W/1 -> IMAPve_g_R1_W_1/1
  IMAPve_d_R1_Type_1/1 -> SignalBusCreator/73(R1_Type)  "IMAPve_d_R1_Type"
  IMAPve_d_R1_Type/1 -> IMAPve_d_R1_Type_1/1
  IMAPve_d_R1_Q_1/1 -> SignalBusCreator/72(R1_Q)  "IMAPve_d_R1_Q"
  IMAPve_d_R1_Q/1 -> IMAPve_d_R1_Q_1/1
  IMAPve_g_R1_VR_1/1 -> SignalBusCreator/71(R1_VR)  "IMAPve_g_R1_VR"
  IMAPve_g_R1_VR/1 -> IMAPve_g_R1_VR_1/1
  IMAPve_g_R1_C3_1/1 -> SignalBusCreator/70(R1_C3)  "IMAPve_g_R1_C3"
  IMAPve_g_R1_C3/1 -> IMAPve_g_R1_C3_1/1
  IMAPve_g_R1_C2_1/1 -> SignalBusCreator/69(R1_C2)  "IMAPve_g_R1_C2"
  IMAPve_g_R1_C2/1 -> IMAPve_g_R1_C2_1/1
  IMAPve_g_R1_C1_1/1 -> SignalBusCreator/68(R1_C1)  "IMAPve_g_R1_C1"
  IMAPve_g_R1_C1/1 -> IMAPve_g_R1_C1_1/1
  IMAPve_g_R1_C0_1/1 -> SignalBusCreator/67(R1_C0)  "IMAPve_g_R1_C0"
  IMAPve_g_R1_C0/1 -> IMAPve_g_R1_C0_1/1
  IMAPve_g_L1_W_1/1 -> SignalBusCreator/66(L1_W)  "IMAPve_g_L1_W"
  IMAPve_g_L1_W/1 -> IMAPve_g_L1_W_1/1
  IMAPve_d_L1_Type_1/1 -> SignalBusCreator/65(L1_Type)  "IMAPve_d_L1_Type"
  IMAPve_d_L1_Type/1 -> IMAPve_d_L1_Type_1/1
  IMAPve_d_L1_Q_1/1 -> SignalBusCreator/64(L1_Q)  "IMAPve_d_L1_Q"
  IMAPve_d_L1_Q/1 -> IMAPve_d_L1_Q_1/1
  IMAPve_g_L1_VR_1/1 -> SignalBusCreator/63(L1_VR)  "IMAPve_g_L1_VR"
  IMAPve_g_L1_VR/1 -> IMAPve_g_L1_VR_1/1
  IMAPve_g_L1_C3_1/1 -> SignalBusCreator/62(L1_C3)  "IMAPve_g_L1_C3"
  IMAPve_g_L1_C3/1 -> IMAPve_g_L1_C3_1/1
  IMAPve_g_L1_C2_1/1 -> SignalBusCreator/61(L1_C2)  "IMAPve_g_L1_C2"
  IMAPve_g_L1_C2/1 -> IMAPve_g_L1_C2_1/1
  IMAPve_g_L1_C1_1/1 -> SignalBusCreator/60(L1_C1)  "IMAPve_g_L1_C1"
  IMAPve_g_L1_C1/1 -> IMAPve_g_L1_C1_1/1
  IMAPve_g_L1_C0_1/1 -> SignalBusCreator/59(L1_C0)  "IMAPve_g_L1_C0"
  IMAPve_g_L1_C0/1 -> IMAPve_g_L1_C0_1/1
  IMAPve_g_R0_W_1/1 -> SignalBusCreator/58(R0_W)  "IMAPve_g_R0_W"
  IMAPve_g_R0_W/1 -> IMAPve_g_R0_W_1/1
  IMAPve_d_R0_Type_1/1 -> SignalBusCreator/57(R0_Type)  "IMAPve_d_R0_Type"
  IMAPve_d_R0_Type/1 -> IMAPve_d_R0_Type_1/1
  IMAPve_d_R0_Q_1/1 -> SignalBusCreator/56(R0_Q)  "IMAPve_d_R0_Q"
  IMAPve_d_R0_Q/1 -> IMAPve_d_R0_Q_1/1
  IMAPve_g_R0_VR_1/1 -> SignalBusCreator/55(R0_VR)  "IMAPve_g_R0_VR"
  IMAPve_g_R0_VR/1 -> IMAPve_g_R0_VR_1/1
  IMAPve_g_R0_C3_1/1 -> SignalBusCreator/54(R0_C3)  "IMAPve_g_R0_C3"
  IMAPve_g_R0_C3/1 -> IMAPve_g_R0_C3_1/1
  IMAPve_g_R0_C2_1/1 -> SignalBusCreator/53(R0_C2)  "IMAPve_g_R0_C2"
  IMAPve_g_R0_C2/1 -> IMAPve_g_R0_C2_1/1
  IMAPve_g_R0_C1_1/1 -> SignalBusCreator/52(R0_C1)  "IMAPve_g_R0_C1"
  IMAPve_g_R0_C1/1 -> IMAPve_g_R0_C1_1/1
  IMAPve_g_R0_C0_1/1 -> SignalBusCreator/51(R0_C0)  "IMAPve_g_R0_C0"
  IMAPve_g_R0_C0/1 -> IMAPve_g_R0_C0_1/1
  IMAPve_g_L0_W_1/1 -> SignalBusCreator/50(L0_W)  "IMAPve_g_L0_W"
  IMAPve_g_L0_W/1 -> IMAPve_g_L0_W_1/1
  IMAPve_d_L0_Type_1/1 -> SignalBusCreator/49(L0_Type)  "IMAPve_d_L0_Type"
  IMAPve_d_L0_Type/1 -> IMAPve_d_L0_Type_1/1
  IMAPve_d_L0_Q_1/1 -> SignalBusCreator/48(L0_Q)  "IMAPve_d_L0_Q"
  IMAPve_d_L0_Q/1 -> IMAPve_d_L0_Q_1/1
  IMAPve_g_L0_VR_1/1 -> SignalBusCreator/47(L0_VR)  "IMAPve_g_L0_VR"
  IMAPve_g_L0_VR/1 -> IMAPve_g_L0_VR_1/1
  IMAPve_g_L0_C3_1/1 -> SignalBusCreator/46(L0_C3)  "IMAPve_g_L0_C3"
  IMAPve_g_L0_C3/1 -> IMAPve_g_L0_C3_1/1
  IMAPve_g_L0_C2_1/1 -> SignalBusCreator/45(L0_C2)  "IMAPve_g_L0_C2"
  IMAPve_g_L0_C2/1 -> IMAPve_g_L0_C2_1/1
  IMAPve_g_L0_C1_1/1 -> SignalBusCreator/44(L0_C1)  "IMAPve_g_L0_C1"
  IMAPve_g_L0_C1/1 -> IMAPve_g_L0_C1_1/1
  IMAPve_g_L0_C0_1/1 -> SignalBusCreator/43(L0_C0)  "IMAPve_g_L0_C0"
  IMAPve_g_L0_C0/1 -> IMAPve_g_L0_C0_1/1
  IMAPve_d_Fusion_Status_1/1 -> SignalBusCreator/42(Fusion_Status)  "IMAPve_d_Fusion_Status"
  IMAPve_d_Fusion_Status/1 -> IMAPve_d_Fusion_Status_1/1
  IMAPve_d_Sensor_Status_1/1 -> SignalBusCreator/41(Sensor_Status)  "IMAPve_d_Sensor_Status"
  IMAPve_d_Sensor_Status/1 -> IMAPve_d_Sensor_Status_1/1
  IMAPve_d_Camera_Status_1/1 -> SignalBusCreator/40(Camera_Status)  "IMAPve_d_Camera_Status"
  IMAPve_d_Camera_Status/1 -> IMAPve_d_Camera_Status_1/1
  IMAPve_d_TCU_TCU_Available_1/1 -> SignalBusCreator/39(TCU_Available)  "IMAPve_d_TCU_TCU_Available"
  IMAPve_d_TCU_TCU_Available/1 -> IMAPve_d_TCU_TCU_Available_1/1
  IMAPve_d_TCU_Actual_Gear_1/1 -> SignalBusCreator/38(TCU_ActualGear)  "IMAPve_d_TCU_Actual_Gear"
  IMAPve_d_TCU_Actual_Gear/1 -> IMAPve_d_TCU_Actual_Gear_1/1
  IMAPve_g_EMS_RealPedal_1/1 -> SignalBusCreator/37(AccPedal_Pos)  "IMAPve_g_EMS_RealPedal"
  IMAPve_g_EMS_RealPedal/1 -> IMAPve_g_EMS_RealPedal_1/1
  IMAPve_d_BCM_RightTurn_Switch_1/1 -> SignalBusCreator/36(BCM_RightTurn_Switch)  "IMAPve_d_BCM_RightTurn_Switch"
  IMAPve_d_BCM_RightTurn_Switch/1 -> IMAPve_d_BCM_RightTurn_Switch_1/1
  IMAPve_d_BCM_LeftTurn_Switch_1/1 -> SignalBusCreator/35(BCM_LeftTurn_Switch)  "IMAPve_d_BCM_LeftTurn_Switch"
  IMAPve_d_BCM_LeftTurn_Switch/1 -> IMAPve_d_BCM_LeftTurn_Switch_1/1
  IMAPve_d_BCM_Right_Light_1/1 -> SignalBusCreator/34(BCM_Right_Light)  "IMAPve_d_BCM_Right_Light"
  IMAPve_d_BCM_Right_Light/1 -> IMAPve_d_BCM_Right_Light_1/1
  IMAPve_d_BCM_Left_Light_1/1 -> SignalBusCreator/33(BCM_Left_Light)  "IMAPve_d_BCM_Left_Light"
  IMAPve_d_BCM_Left_Light/1 -> IMAPve_d_BCM_Left_Light_1/1
  IMAPve_d_BCM_HazardLamp_1/1 -> SignalBusCreator/32(BCM_Double_Light)  "IMAPve_d_BCM_HazardLamp"
  IMAPve_d_BCM_HazardLamp/1 -> IMAPve_d_BCM_HazardLamp_1/1
  IMAPve_d_ESC_VehSpd_Valid_1/1 -> SignalBusCreator/31(ESC_VehSpd_Valid)  "IMAPve_d_ESC_VehSpd_Valid"
  IMAPve_d_ESC_VehSpd_Valid/1 -> IMAPve_d_ESC_VehSpd_Valid_1/1
  IMAPve_g_ESC_Brake_Press_1/1 -> SignalBusCreator/30(ESC_Brake_Press)  "IMAPve_g_ESC_Brake_Press"
  IMAPve_g_ESC_Brake_Press/1 -> IMAPve_g_ESC_Brake_Press_1/1
  IMAPve_d_ESC_LonAcc_Valid_1/1 -> SignalBusCreator/29(ESC_LonAcc_Valid)  "IMAPve_d_ESC_LonAcc_Valid"
  IMAPve_d_ESC_LonAcc_Valid/1 -> IMAPve_d_ESC_LonAcc_Valid_1/1
  IMAPve_g_ESC_LonAcc_1/1 -> SignalBusCreator/28(ESC_LonAcc)  "IMAPve_g_ESC_LonAcc"
  IMAPve_g_ESC_LonAcc/1 -> IMAPve_g_ESC_LonAcc_1/1
  IMAPve_g_ESC_VehSpd_1/1 -> SignalBusCreator/27(ESC_VehSpd)  "IMAPve_g_ESC_VehSpd"
  IMAPve_g_ESC_VehSpd/1 -> IMAPve_g_ESC_VehSpd_1/1
  IMAPve_g_ESC_UnYawRate_1/1 -> SignalBusCreator/26(ESC_UnYawRate)  "IMAPve_g_ESC_UnYawRate"
  IMAPve_g_ESC_UnYawRate/1 -> IMAPve_g_ESC_UnYawRate_1/1
  IMAPve_d_ESC_YawRate_Valid_1/1 -> SignalBusCreator/25(ESC_YawRate_Valid)  "IMAPve_d_ESC_YawRate_Valid"
  IMAPve_d_ESC_YawRate_Valid/1 -> IMAPve_d_ESC_YawRate_Valid_1/1
  IMAPve_g_ESC_YawRate_1/1 -> SignalBusCreator/24(ESC_YawRate)  "IMAPve_g_ESC_YawRate"
  IMAPve_g_ESC_YawRate/1 -> IMAPve_g_ESC_YawRate_1/1
  IMAPve_d_ESC_LatAcc_Valid_1/1 -> SignalBusCreator/23(ESC_LatAcc_Valid)  "IMAPve_d_ESC_LatAcc_Valid"
  IMAPve_d_ESC_LatAcc_Valid/1 -> IMAPve_d_ESC_LatAcc_Valid_1/1
  IMAPve_g_ESC_LatAcc_1/1 -> SignalBusCreator/22(ESC_LatAcc)  "IMAPve_g_ESC_LatAcc"
  IMAPve_g_ESC_LatAcc/1 -> IMAPve_g_ESC_LatAcc_1/1
  IMAPve_g_SW_Angle_Speed_1/1 -> SignalBusCreator/21(SW_Angle_Speed)  "IMAPve_g_SW_Angle_Speed"
  IMAPve_g_SW_Angle_Speed/1 -> IMAPve_g_SW_Angle_Speed_1/1
  IMAPve_g_SW_Angle_1/1 -> SignalBusCreator/20(SW_Angle)  "IMAPve_g_SW_Angle"
  IMAPve_g_SW_Angle/1 -> IMAPve_g_SW_Angle_1/1
  IMAPve_g_EPS_SteeringAngle_1/1 -> SignalBusCreator/19(EPS_SteeringAngle)  "IMAPve_g_EPS_SteeringAngle"
  IMAPve_g_EPS_SteeringAngle/1 -> IMAPve_g_EPS_SteeringAngle_1/1
  IMAPve_d_EPS_SteeringAngle_Flag_1/1 -> SignalBusCreator/18(EPS_SteeringAngle_Flag)  "IMAPve_d_EPS_SteeringAngle_Flag"
  IMAPve_d_EPS_SteeringAngle_Flag/1 -> IMAPve_d_EPS_SteeringAngle_Flag_1/1
  IMAPve_d_EPS_ESA_State_1/1 -> SignalBusCreator/17(EPS_ESA_State)  "IMAPve_d_EPS_ESA_State"
  IMAPve_d_EPS_ESA_State/1 -> IMAPve_d_EPS_ESA_State_1/1
  IMAPve_d_EPS_Driver_Override_1/1 -> SignalBusCreator/16(EPS_Driver_Override)  "IMAPve_d_EPS_Driver_Override"
  IMAPve_d_EPS_Driver_Override/1 -> IMAPve_d_EPS_Driver_Override_1/1
  IMAPve_d_EPS_Steer_Hold_State_1/1 -> SignalBusCreator/15(EPS_SWHold_State)  "IMAPve_d_EPS_Steer_Hold_State"
  IMAPve_d_EPS_Steer_Hold_State/1 -> IMAPve_d_EPS_Steer_Hold_State_1/1
  IMAPve_g_EPS_LKA_Current_1/1 -> SignalBusCreator/14(EPS_LKA_Current)  "IMAPve_g_EPS_LKA_Current"
  IMAPve_g_EPS_LKA_Current/1 -> IMAPve_g_EPS_LKA_Current_1/1
  IMAPve_d_EPS_TrqLim_State_1/1 -> SignalBusCreator/13(EPS_TrqLim_State)  "IMAPve_d_EPS_TrqLim_State"
  IMAPve_d_EPS_TrqLim_State/1 -> IMAPve_d_EPS_TrqLim_State_1/1
  IMAPve_d_SWS_Failure_Status_1/1 -> SignalBusCreator/12(SWS_Failure_Status)  "IMAPve_d_SWS_Failure_Status"
  IMAPve_d_SWS_Failure_Status/1 -> IMAPve_d_SWS_Failure_Status_1/1
  IMAPve_d_SAS_Trim_State_1/1 -> SignalBusCreator/11(SAS_Trim_State)  "IMAPve_d_SAS_Trim_State"
  IMAPve_d_SAS_Trim_State/1 -> IMAPve_d_SAS_Trim_State_1/1
  IMAPve_d_SAS_Clb_State_1/1 -> SignalBusCreator/10(SAS_Clb_State)  "IMAPve_d_SAS_Clb_State"
  IMAPve_d_SAS_Clb_State/1 -> IMAPve_d_SAS_Clb_State_1/1
  IMAPve_d_EPS_Trq_State_1/1 -> SignalBusCreator/9(EPS_Trq_State)  "IMAPve_d_EPS_Trq_State"
  IMAPve_d_EPS_Trq_State/1 -> IMAPve_d_EPS_Trq_State_1/1
  IMAPve_g_EPS_SW_Trq_1/1 -> SignalBusCreator/8(EPS_SW_Trq)  "IMAPve_g_EPS_SW_Trq"
  IMAPve_g_EPS_SW_Trq/1 -> IMAPve_g_EPS_SW_Trq_1/1
  IMAPve_d_EPS_LKA_State_1/1 -> SignalBusCreator/7(EPS_LKA_State)  "IMAPve_d_EPS_LKA_State"
  IMAPve_d_EPS_LKA_State/1 -> IMAPve_d_EPS_LKA_State_1/1
  IMAPve_d_MP5_Work_State_1/1 -> SignalBusCreator/6(MP5_Work_State)  "IMAPve_d_MP5_Work_State"
  IMAPve_d_MP5_Work_State/1 -> IMAPve_d_MP5_Work_State_1/1
  IMAPve_d_APA_AutoPark_WorkSt_1/1 -> SignalBusCreator/5(APA_AutoPark_WorkSt)  "IMAPve_d_APA_AutoPark_WorkSt"
  IMAPve_d_APA_AutoPark_WorkSt/1 -> IMAPve_d_APA_AutoPark_WorkSt_1/1
  IMAPve_d_LDW_Warn_Mode_1/1 -> SignalBusCreator/4(LDW_Warn_Mode)  "IMAPve_d_LDW_Warn_Mode"
  IMAPve_d_LDW_Warn_Mode/1 -> IMAPve_d_LDW_Warn_Mode_1/1
  IMAPve_d_LKA_Mode_1/1 -> SignalBusCreator/3(LKA_Mode)  "IMAPve_d_LKA_Mode"
  IMAPve_d_LKA_Mode/1 -> IMAPve_d_LKA_Mode_1/1
  IMAPve_d_LKA_Main_Switch_1/1 -> SignalBusCreator/2(LKA_Main_Switch)  "IMAPve_d_LKA_Main_Switch"
  IMAPve_d_LKA_Main_Switch/1 -> IMAPve_d_LKA_Main_Switch_1/1
  FDMMve_d_LkaFcnConf_1/1 -> SignalBusCreator/1(LkaFcnConf)  "FDMMve_d_LkaFcnConf"
  FDMMve_d_LkaFcnConf/1 -> FDMMve_d_LkaFcnConf_1/1

== system LKAS_AutoSave_DF_20211126_SW5/LKAS/LL ==
  bsInInfo : Inport
  bsLLClb : Inport  Port=2
  Bus Selector : BusSelector  OutputSignals=bsMP5Info.LKA_Mode
  Bus Selector1 : BusSelector  OutputSignals=bsLaneInfo.bsR0Info.R0_Q,bsLaneInfo.bsL0Info.L0_Q
  Bus Selector2 : BusSelector  OutputSignals=bsEPSInfo
  Bus Selector3 : BusSelector  OutputSignals=LKA_State,LDW_State
  Bus Selector4 : BusSelector  OutputSignals=bsLaneInfo.Fusion_AdditionalInf.Carema_Status
  Bus Selector5 : BusSelector  OutputSignals=bsMP5Info.LKA_Mode
  Fault_Diagnostic : Subsystem
  Ground1 : Ground
  Ground3 : Ground
  Human Machine Interface (HMI) : Subsystem
  LL Inputs Mapping : Subsystem
  LLOn : Subsystem
  LLOut : Subsystem
  Terminator : Terminator
  Version : Constant  Value=211116  OutMin=20410  OutMax=220630  OutDataTypeStr=single
  LL_bsLLOut : Outport
      settings: AttributesFormatString=Disable Action: %<OutputWhenDisabled>
  tag scope: LLMon=global
  wires:
  [bsSignalFault] -> LLOn/3(bsSignalFault)
  [bsLLClb] -> LLOn/2(bsLLClb)
  [bsInfo] -> LLOn/1(bsInInfo), Bus Selector/1
  [bsInInfo] -> LL Inputs Mapping/1(bsInInfo)
  LL Inputs Mapping/1(bsInfo) -> [bsInfo]
  [bsInInfo] -> Fault_Diagnostic/1(bsInInfo)
  Fault_Diagnostic/1(bsSignalFault) -> [bsSignalFault]
  LLOn/5(LLMon) -> [LLMon]
  LLOn/4(M) -> [LLOn_M]
  LLOn/3(phiSWACmd) -> [LLOn_phiSWACmd]
  LLOn/1(bsLLState) -> [LLOn_bsLLState]
  bsLLClb/1 -> [bsLLClb]
  LLOn/2(LDW_Flag) -> [LLOn_bsLDWWarnInfo]
  Version/1 -> Terminator/1  "ob_LKA_Version"
  Human Machine Interface (HMI)/1(HMI_LDWLKA) -> [HMI_bsLLHMI]  "bsLLHMI"
  bsInInfo/1 -> [bsInInfo]
  Bus Selector/1 -> LLOn/Enable  "<LKA_Mode>"
  [HMI_bsLLHMI] -> LLOut/3(LLOut_bsLLHMI)
  LLOut/1(LL_bsLLOut) -> LL_bsLLOut/1
  [LLOn_bsLLState] -> LLOut/1(LLOut_bsLLState)
  [LLOn_M] -> LLOut/4(LLOut_M)
  [bsInfo] -> LLOut/5(LLOut_bsInfo)
  [LLOn_phiSWACmd] -> LLOut/2(LLOut_phiSWACmd)
  [bsInfo] -> Bus Selector4/1, Bus Selector2/1, Bus Selector1/1, Bus Selector5/1
  Bus Selector3/2 -> Human Machine Interface (HMI)/3(HMI_LDW_STATE)  "<LDW_State>"
  Bus Selector3/1 -> Human Machine Interface (HMI)/2(HMI_LKA_STATE)  "<LKA_State>"
  Ground3/1 -> Human Machine Interface (HMI)/10(HMI_stFaultCSyn)
  Ground1/1 -> Human Machine Interface (HMI)/8(HMI_camera_common_fault)
  Bus Selector4/1 -> Human Machine Interface (HMI)/9(HMI_Front_Camera_Blocked)  "<Carema_Status>"
  [LLOn_bsLLState] -> Bus Selector3/1
  Bus Selector5/1 -> Human Machine Interface (HMI)/1(HMI_stDACmode)  "<LKA_Mode>"
  Bus Selector1/1 -> Human Machine Interface (HMI)/5(HMI_R0_Quality)  "<R0_Q>"
  Bus Selector1/2 -> Human Machine Interface (HMI)/6(HMI_L0_Quality)  "<L0_Q>"
  Bus Selector2/1 -> Human Machine Interface (HMI)/7(HMI_EPSInfo)  "<bsEPSInfo>"
  [LLOn_bsLDWWarnInfo] -> Human Machine Interface (HMI)/4(HMI_LDWWarn)

== system LKAS_AutoSave_DF_20211126_SW5/LKAS/LLClb ==
  Bus Creator : BusCreator  Inputs=4
  ConstantClb : Subsystem
  LDWClb : Subsystem
  LKAClb : Subsystem
  LLSMConClb : Subsystem
  LLClb_bsLLClb : Outport
  wires:
  LKAClb/1(LKAClb) -> Bus Creator/3  "bsLKAClb"
  LDWClb/1(LDWClb) -> Bus Creator/2  "bsLDWClb"
  Bus Creator/1 -> LLClb_bsLLClb/1  "bsLLClb"
  LLSMConClb/1(LLSMConClb) -> Bus Creator/1  "bsLLSMConClb"
  ConstantClb/1(ConstantClb) -> Bus Creator/4  "bsConstantClb"
